simulink model "extendidoAkermanBernulliSeguimientoExtendido"  (R2023a)
settings: Solver=ode4  StartTime=0.0  StopTime=160  FixedStep=0.001  RelTol=1e-3
settings Model: Creator=uriel  LastModifiedBy=uriel

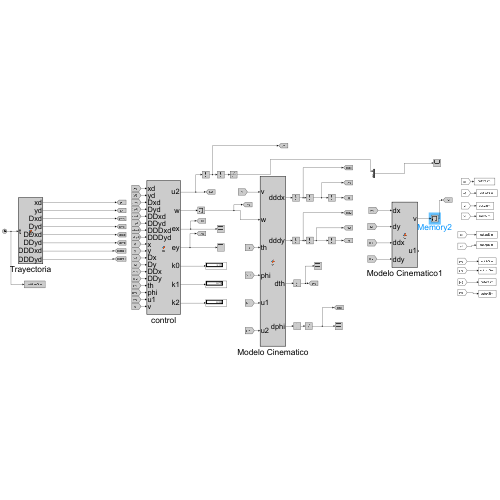
[thumbnail: Simulink's stored preview of the top-level diagram]
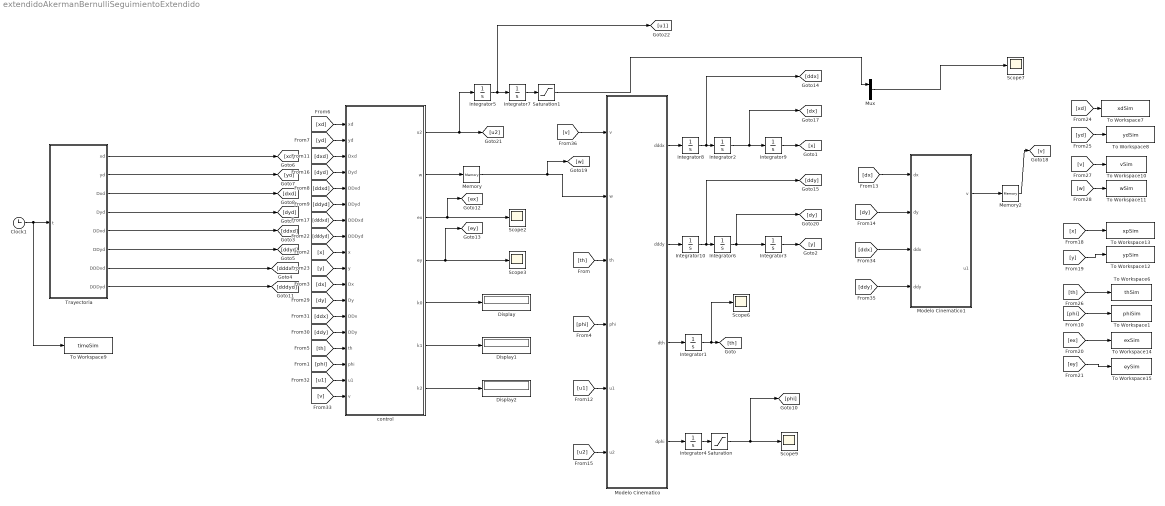
== system extendidoAkermanBernulliSeguimientoExtendido ==
  Clock1 : Clock
  Display : Display
  Display1 : Display
  Display2 : Display
  Integrator1 : Integrator  InitialCondition=1.6836170254102722
  Integrator{2,4..5,7..8,10} (6 alike) : Integrator
  Integrator3 : Integrator  InitialCondition=-0.06034485623240471
  Integrator6 : Integrator  InitialCondition=0.1
  Integrator9 : Integrator  InitialCondition=2.5263853073120117
  Memory : Memory
  Memory2 : Memory  InitialCondition=0.07
  Modelo Cinematico : MATLAB Function  TreatAsAtomicUnit=on
  Modelo Cinematico1 : MATLAB Function  TreatAsAtomicUnit=on
  Mux : Mux  Inputs=2
  Saturation : Saturate  UpperLimit=0.38  LowerLimit=-0.4
  Saturation1 : Saturate  UpperLimit=1.0  LowerLimit=0.1
  Scope{2..3,6..7,9} (5 alike) : Scope
  To Workspace1 : ToWorkspace  VariableName=phiSim  SaveFormat=Structure  SampleTime=-1
  To Workspace10 : ToWorkspace  VariableName=vSim  SaveFormat=Structure  SampleTime=-1
  To Workspace11 : ToWorkspace  VariableName=wSim  SaveFormat=Structure  SampleTime=-1
  To Workspace12 : ToWorkspace  VariableName=ypSim  SaveFormat=Structure  SampleTime=-1
  To Workspace13 : ToWorkspace  VariableName=xpSim  SaveFormat=Structure  SampleTime=-1
  To Workspace14 : ToWorkspace  VariableName=exSim  SaveFormat=Structure  SampleTime=-1
  To Workspace15 : ToWorkspace  VariableName=eySim  SaveFormat=Structure  SampleTime=-1
  To Workspace6 : ToWorkspace  VariableName=thSim  SaveFormat=Structure  SampleTime=-1
  To Workspace7 : ToWorkspace  VariableName=xdSim  SaveFormat=Structure  SampleTime=-1
  To Workspace8 : ToWorkspace  VariableName=ydSim  SaveFormat=Structure  SampleTime=-1
  To Workspace9 : ToWorkspace  VariableName=timeSim  SaveFormat=Structure  SampleTime=-1
  Trayectoria : MATLAB Function  TreatAsAtomicUnit=on
  control : MATLAB Function  TreatAsAtomicUnit=on
  wires:
  Trayectoria/3(Dxd) -> [dxd]
  Trayectoria/2(yd) -> [yd]
  Clock1/1 -> To Workspace9/1, Trayectoria/1(t)
  Trayectoria/1(xd) -> [xd]
  Trayectoria/8(DDDyd) -> [dddyd]
  Trayectoria/7(DDDxd) -> [dddxd]
  Trayectoria/6(DDyd) -> [ddyd]
  Trayectoria/5(DDxd) -> [ddxd]
  Trayectoria/4(Dyd) -> [dyd]
  [phi] -> To Workspace1/1
  [v] -> control/18(v)
  Integrator2/1 -> [dx], Integrator9/1
  [dx] -> control/11(Dx)
  Modelo Cinematico1/1(v) -> Memory2/1
  Integrator8/1 -> [ddx], Integrator2/1
  [phi] -> control/16(phi)
  Memory/1 -> [w], Modelo Cinematico/2(w)
  [xd] -> To Workspace7/1
  [yd] -> To Workspace8/1
  [w] -> To Workspace11/1
  [th] -> To Workspace6/1
  [v] -> To Workspace10/1
  [y] -> control/10(y)
  [x] -> control/9(x)
  [ddyd] -> control/6(DDyd)
  [x] -> To Workspace13/1
  [ey] -> To Workspace15/1
  [u1] -> control/17(u1)
  [dyd] -> control/4(Dyd)
  [phi] -> Modelo Cinematico/4(phi)
  control/6(k1) -> Display1/1
  [ddxd] -> control/5(DDxd)
  Integrator5/1 -> [u1], Integrator7/1
  control/5(k0) -> Display/1
  Modelo Cinematico/1(dddx) -> Integrator8/1
  [ex] -> To Workspace14/1
  control/2(w) -> Memory/1
  Integrator6/1 -> [dy], Integrator3/1
  [u2] -> Modelo Cinematico/6(u2)
  [dddxd] -> control/7(DDDxd)
  [ddy] -> Modelo Cinematico1/4(ddy)
  Modelo Cinematico/4(dphi) -> Integrator4/1
  [v] -> Modelo Cinematico/1(v)
  [th] -> Modelo Cinematico/3(th)
  Mux/1 -> Scope7/1
  [y] -> To Workspace12/1
  Integrator7/1 -> Saturation1/1
  [dddyd] -> control/8(DDDyd)
  [dx] -> Modelo Cinematico1/1(dx)
  Integrator10/1 -> [ddy], Integrator6/1
  control/1(u2) -> Integrator5/1, [u2]
  [dxd] -> control/3(Dxd)
  [u1] -> Modelo Cinematico/5(u1)
  Modelo Cinematico/2(dddy) -> Integrator10/1
  control/7(k2) -> Display2/1
  [ddx] -> control/13(DDx)
  [xd] -> control/1(xd)
  [ddy] -> control/14(DDy)
  [dy] -> control/12(Dy)
  Integrator1/1 -> Scope6/1, [th]
  [dy] -> Modelo Cinematico1/2(dy)
  control/3(ex) -> [ex], Scope2/1
  Saturation/1 -> Scope9/1, [phi]
  [ddx] -> Modelo Cinematico1/3(ddx)
  Integrator9/1 -> [x]
  Integrator4/1 -> Saturation/1
  control/4(ey) -> Scope3/1, [ey]
  Integrator3/1 -> [y]
  [yd] -> control/2(yd)
  [th] -> control/15(th)
  Modelo Cinematico/3(dth) -> Integrator1/1
  Memory2/1 -> [v]
  Saturation1/1 -> Mux/1

== matlab function extendidoAkermanBernulliSeguimientoExtendido/Modelo Cinematico1 ==
  data: dx input; dy input; v output; ddx input; ddy input; u1 output
function [v,u1]  = fcn(dx,dy,ddx,ddy)

%%%%%%%%%%%%%% MATRIZ DE DESACOPLAMIENTO %%%%%%%%%%%%%%%%%%%%%55
v=sqrt(dx*dx+dy*dy);
u1=sqrt(ddx*ddx+ddy*ddy);

== matlab function extendidoAkermanBernulliSeguimientoExtendido/Modelo Cinematico ==
  data: v input; w input; dddx output; th input; dddy output; dth output; phi input; dphi output; u1 input; u2 input
function [dddx,dddy,dth,dphi]  = fcn(v,w,th,phi,u1, u2)
l=0.26;

%% Matriz de desacoplamiento
A=[cos(th), -v*v*sin(th)*(1+(tan(phi)*tan(phi)))/l;
   sin(th),  v*v*cos(th)*(1+(tan(phi)*tan(phi)))/l];
%% Matriz de compensanción
B=[-(3*v*u1*sin(th)*tan(phi)/l)-v*v*v*cos(th)*tan(phi)*tan(phi)/(l*l);
   (3*v*u1*cos(th)*tan(phi)/l)-v*v*v*sin(th)*tan(phi)*tan(phi)/(l*l)];

U = [u2;w];
DDDz = A*U+B;

dddx = DDDz(1);
dddy = DDDz(2);
dth=v*tan(phi)/l;
dphi=w;

== matlab function extendidoAkermanBernulliSeguimientoExtendido/Trayectoria ==
  data: xd output; yd output; Dxd output; Dyd output; DDxd output; DDyd output; DDDxd output; t input; DDDyd output
function [xd,yd,Dxd,Dyd,DDxd,DDyd,DDDxd,DDDyd]   = fcn(t)
T=80;
f=1/T;
w=2*pi*f;
a = 2.5;
d = 3.0;

xd = a*cos(w*t)/(1+(sin(w*t)*(sin(w*t))));
Dxd = -a*((w*sin(w*t)/(1+sin(w*t)*sin(w*t)))+2*w*sin(w*t)*cos(w*t)*cos(w*t)/((1+(sin(w*t)*sin(w*t)))*(1+(sin(w*t)*sin(w*t)))));
DDxd = a*(-(w*w*cos(w*t)/(1+sin(w*t)*sin(w*t)))+(6*w*w*sin(w*t)*sin(w*t)*cos(w*t)/((1+sin(w*t)*sin(w*t))*(1+sin(w*t)*sin(w*t))))-(2*w*w*cos(w*t)*cos(w*t)*cos(w*t)/((1+sin(w*t)*sin(w*t))*(1+sin(w*t)*sin(w*t))))+(8*w*w*sin(w*t)*sin(w*t)*cos(w*t)*cos(w*t)*cos(w*t)/((1+sin(w*t)*sin(w*t))*(1+sin(w*t)*sin(w*t))*(1+sin(w*t)*sin(w*t)))));
DDDxd = a*((w*w*w*sin(w*t)/(1+sin(w*t)*sin(w*t)))+(20*w*w*w*sin(w*t)*cos(w*t)*cos(w*t)/((1+sin(w*t)*sin(w*t))*(1+sin(w*t)*sin(w*t))))-(6*w*w*w*sin(w*t)*sin(w*t)*sin(w*t)/((1+sin(w*t)*sin(w*t))*(1+sin(w*t)*sin(w*t))))-(48*w*w*w*sin(w*t)*sin(w*t)*sin(w*t)*cos(w*t)*cos(w*t)/((1+sin(w*t)*sin(w*t))*(1+sin(w*t)*sin(w*t))*(1+sin(w*t)*sin(w*t))))+(24*w*w*w*sin(w*t)*cos(w*t)*cos(w*t)*cos(w*t)*cos(w*t)/((1+sin(w*t)*sin(w*t))*(1+sin(w*t)*sin(w*t))*(1+sin(w*t)*sin(w*t))))-(48*w*w*w*sin(w*t)*sin(w*t)*sin(w*t)*cos(w*t)*cos(w*t)*cos(w*t)*cos(w*t)/((1+sin(w*t)*sin(w*t))*(1+sin(w*t)*sin(w*t))*(1+sin(w*t)*sin(w*t))*(1+sin(w*t)*sin(w*t)))));

yd = d*(sin(w*t)*cos(w*t))/(1+(sin(w*t)*sin(w*t)));
Dyd = d*((w*cos(w*t)*cos(w*t)/(1+sin(w*t)*sin(w*t)))-(w*sin(w*t)*sin(w*t)/(1+sin(w*t)*sin(w*t)))-(2*w*sin(w*t)*sin(w*t)*cos(w*t)*cos(w*t)/((1+sin(w*t)*sin(w*t))*(1+sin(w*t)*sin(w*t)))));
DDyd = d*((-4*w*w*sin(w*t)*cos(w*t)/(1+sin(w*t)*sin(w*t)))-(6*w*w*sin(w*t)*cos(w*t)*cos(w*t)*cos(w*t)/((1+sin(w*t)*sin(w*t))*(1+sin(w*t)*sin(w*t))))+(6*w*w*sin(w*t)*sin(w*t)*sin(w*t)*cos(w*t)/((1+sin(w*t)*sin(w*t))*(1+sin(w*t)*sin(w*t))))+(8*w*w*sin(w*t)*sin(w*t)*sin(w*t)*cos(w*t)*cos(w*t)*cos(w*t)/((1+sin(w*t)*sin(w*t))*(1+sin(w*t)*sin(w*t))*(1+sin(w*t)*sin(w*t)))));
DDDyd = d*((-4*w*w*w*cos(w*t)*cos(w*t)/(1+sin(w*t)*sin(w*t)))+(4*w*w*w*sin(w*t)*sin(w*t)/(1+sin(w*t)*sin(w*t)))+(44*w*w*w*sin(w*t)*sin(w*t)*cos(w*t)*cos(w*t)/((1+sin(w*t)*sin(w*t))*(1+sin(w*t)*sin(w*t))))-(6*w*w*w*cos(w*t)*cos(w*t)*cos(w*t)*cos(w*t)/((1+sin(w*t)*sin(w*t))*(1+sin(w*t)*sin(w*t))))-(6*w*w*w*sin(w*t)*sin(w*t)*sin(w*t)*sin(w*t)/((1+sin(w*t)*sin(w*t))*(1+sin(w*t)*sin(w*t))))+(48*w*w*w*sin(w*t)*sin(w*t)*cos(w*t)*cos(w*t)*cos(w*t)*cos(w*t)/((1+sin(w*t)*sin(w*t))*(1+sin(w*t)*sin(w*t))*(1+sin(w*t)*sin(w*t))))-(48*w*w*w*sin(w*t)*sin(w*t)*sin(w*t)*sin(w*t)*cos(w*t)*cos(w*t)/((1+sin(w*t)*sin(w*t))*(1+sin(w*t)*sin(w*t))*(1+sin(w*t)*sin(w*t))))-(48*w*w*w*sin(w*t)*sin(w*t)*sin(w*t)*sin(w*t)*cos(w*t)*cos(w*t)*cos(w*t)*cos(w*t)/((1+sin(w*t)*sin(w*t))*(1+sin(w*t)*sin(w*t))*(1+sin(w*t)*sin(w*t))*(1+sin(w*t)*sin(w*t)))));

== matlab function extendidoAkermanBernulliSeguimientoExtendido/control ==
  data: u2 output; xd input; yd input; Dxd input; Dyd input; DDxd input; DDyd input; DDDxd input; DDDyd input; x input; y input; Dx input; Dy input; DDx input; DDy input; th input; phi input; w output; ex output; ey output; u1 input; v input; k0 output; k1 output; k2 output
function [u2,w,ex,ey,k0,k1,k2 ]   = fcn(xd,yd,Dxd,Dyd,DDxd,DDyd,DDDxd,DDDyd,x,y,Dx,Dy,DDx,DDy,th,phi,u1,v)
l=0.26;
%% Matriz de desacoplamiento
A=[cos(th), -v*v*sin(th)*(1+(tan(phi)*tan(phi)))/l;
    sin(th),  v*v*cos(th)*(1+(tan(phi)*tan(phi)))/l];
%% Matriz de compensanción
B=[-(3*v*u1*sin(th)*tan(phi)/l)-v*v*v*cos(th)*tan(phi)*tan(phi)/(l*l);
    (3*v*u1*cos(th)*tan(phi)/l)-v*v*v*sin(th)*tan(phi)*tan(phi)/(l*l)];
%% Señales de error
ex = x-xd;
ey = y-yd;
Dex = Dx-Dxd;
Dey = Dy-Dyd;
DDex = DDx-DDxd;
DDey = DDy-DDyd;
% Ganancias de control
ts=6;

z = 1.0;
wn = 4/(ts*z);
p2=2*z*wn;
p3=wn*wn;
p1=7.0;
k0 = p1*p3;
k1 = p3+p1*p2;
k2 = p1+p2;

% kx0 = 3;
% kx1 = 2;
% kx2 = 1;
% ky0 = 3;
% ky1 = 2;
% ky2 = 1;
%% Control auxiliar
rx=-k0*ex-k1*Dex-k2*DDex+DDDxd;
ry=-k0*ey-k1*Dey-k2*DDey+DDDyd;
r=[rx;ry];

%% Control
U=A\(r-B);
u2 = U(1);
w = U(2);
